simulink library "conversionLibrary"  (R2023a)
settings: Solver=VariableStepAuto  StartTime=0.0  StopTime=10.0  RelTol=1e-3
settings Model: Creator=MY PC  LastModifiedBy=MY PC

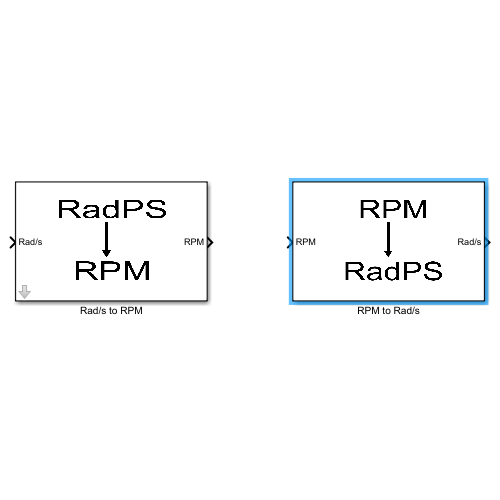
[thumbnail: Simulink's stored preview of the top-level diagram]
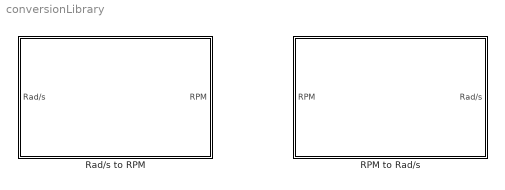
== system conversionLibrary ==
  RPM to Rad/s : Subsystem
      mask Display: image('C:\Users\MY PC\Documents\MATLAB\MATLAB for Engineers\Modelling and Simulation with Simulink\Modeling and Simulation with Simulink\M4\Custom Libraries\RPM2RadPS.png'); % Use "Edit Image" on toolstrip to change.
  Rad/s to RPM : Subsystem
      mask DialogControl DescTextVar Prompt: Converts Rad/s to RPM
      mask Display: image('C:\Users\MY PC\Documents\MATLAB\MATLAB for Engineers\Modelling and Simulation with Simulink\Modeling and Simulation with Simulink\M4\Custom Libraries\RadPS2RPM.png'); % Use "Edit Image" on toolstrip to change.

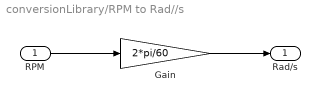
== system conversionLibrary/RPM to Rad//s ==
  RPM : Inport
  Gain : Gain  Gain=2*pi/60
  Rad/s : Outport
  wires:
  RPM/1 -> Gain/1
  Gain/1 -> Rad/s/1

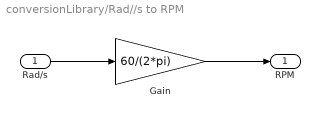
== system conversionLibrary/Rad//s to RPM ==
  Rad/s : Inport
  Gain : Gain  Gain=60/(2*pi)
  RPM : Outport
  wires:
  Rad/s/1 -> Gain/1
  Gain/1 -> RPM/1
